simulink model "deltau_control_pid"  (R2016a)
settings: Solver=VariableStepAuto  StartTime=0.0  StopTime=1000.0  RelTol=1e-3
libraries: simulink x1
settings Model: Creator=win10  LastModifiedBy=Maha

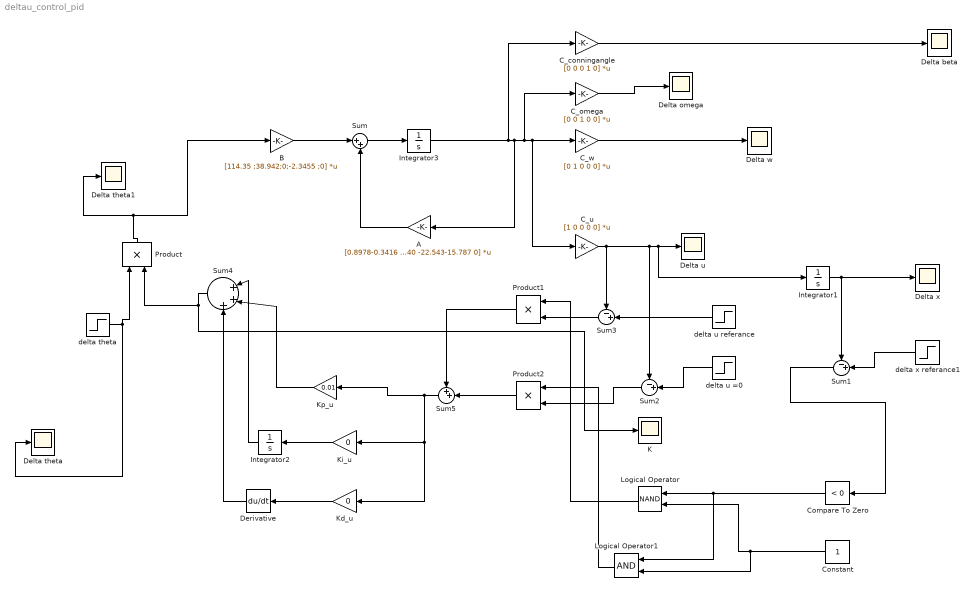
== system deltau_control_pid ==
  A : Gain  Gain=[0.8978-0.3416 1.6108-0.4431 0 0 0 ;0 0 0.2237-0.0318 -17.695-23.318 0 ;0 0 -2.2649-0.5876 1231.1-219.49 0 ;0 0 -0.0063-0.0008 0 0;0.5628-0.2050 0 0.0872-0.0540 -22.543-15.787 0]  Multiplication=Matrix(K*u)
  B : Gain  Gain=[114.35 ;38.942;0;-2.3455 ;0]  Multiplication=Matrix(K*u)
  C_conningangle : Gain  Gain=[0 0 0 1 0]  Multiplication=Matrix(K*u)
  C_omega : Gain  Gain=[0 0 1 0 0]  Multiplication=Matrix(K*u)
  "C_u " : Gain  Gain=[1 0 0 0 0]  Multiplication=Matrix(K*u)
  C_w : Gain  Gain=[0 1 0 0 0]  Multiplication=Matrix(K*u)
  Compare To Zero : simulink/Logic and Bit Operations/Compare To Zero  relop=<  OutDataTypeStr=boolean
  Constant : Constant
  Delta beta : Scope
  Delta omega : Scope
  Delta theta : Scope
  Delta theta1 : Scope
  Delta u : Scope
  Delta w : Scope
  Delta x : Scope
  Derivative : Derivative
  Integrator1 : Integrator
  Integrator2 : Integrator
  Integrator3 : Integrator
  K : Scope
  "Kd_u " : Gain  Gain=0
  "Ki_u " : Gain  Gain=0
  "Kp_u " : Gain  Gain=0.01
  Logical Operator : Logic  Operator=NAND  AllPortsSameDT=off  OutDataTypeStr=boolean
  Logical Operator1 : Logic  AllPortsSameDT=off  OutDataTypeStr=boolean
  Product : Product
  Product1 : Product
  Product2 : Product
  Sum : Sum  Inputs=|++
  Sum1 : Sum  Inputs=-+|
  Sum2 : Sum  Inputs=-+|
  Sum3 : Sum  Inputs=-+|
  Sum4 : Sum  Inputs=|+++
  Sum5 : Sum  Inputs=++|
  delta theta : Step  After=10  SampleTime=1
  delta u =0 : Step  Time=0  After=0  SampleTime=1
  delta u referance : Step  Time=0  After=2  SampleTime=1
  delta x referance1 : Step  Time=0  After=100  SampleTime=1
  wires:
  Integrator3/1 -> C_conningangle/1, A/1, C_omega/1, "C_u "/1, C_w/1
  A/1 -> Sum/2
  B/1 -> Sum/1
  Sum/1 -> Integrator3/1
  C_omega/1 -> Delta omega/1
  C_conningangle/1 -> Delta beta/1
  Sum4/1 -> K/1, Product/2
  delta theta/1 -> Product/1, Delta theta/1
  Product/1 -> B/1, Delta theta1/1
  C_w/1 -> Delta w/1
  "C_u "/1 -> Delta u/1, Integrator1/1, Sum2/1, Sum3/1
  "Ki_u "/1 -> Integrator2/1
  delta u referance/1 -> Sum3/2
  "Kd_u "/1 -> Derivative/1
  "Kp_u "/1 -> Sum4/2
  Integrator2/1 -> Sum4/1
  Derivative/1 -> Sum4/3
  Integrator1/1 -> Delta x/1, Sum1/1
  delta x referance1/1 -> Sum1/2
  Sum1/1 -> Compare To Zero/1
  Compare To Zero/1 -> Logical Operator1/1, Logical Operator/1
  Constant/1 -> Logical Operator1/2, Logical Operator/2
  delta u =0/1 -> Sum2/2
  Sum3/1 -> Product1/2
  Sum2/1 -> Product2/2
  Logical Operator/1 -> Product1/1
  Logical Operator1/1 -> Product2/1
  Product2/1 -> Sum5/2
  Product1/1 -> Sum5/1
  Sum5/1 -> "Kd_u "/1, "Ki_u "/1, "Kp_u "/1
